simulink model "PID_controlinput"  (R2022a)
settings: Solver=VariableStepAuto  StartTime=0.0  StopTime=100  RelTol=1e-3
libraries: cstblocks x2
settings Model: Creator=Linxi Ren  LastModifiedBy=Linxi Ren

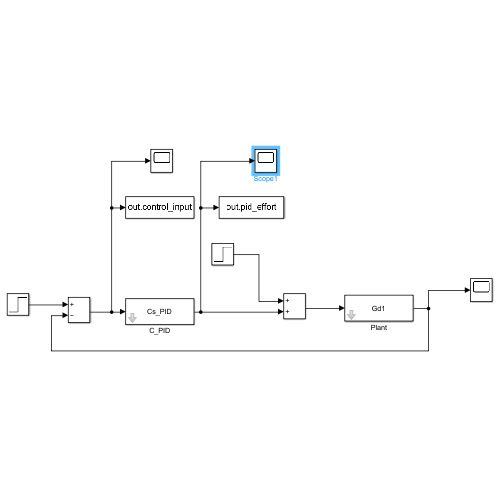
[thumbnail: Simulink's stored preview of the top-level diagram]
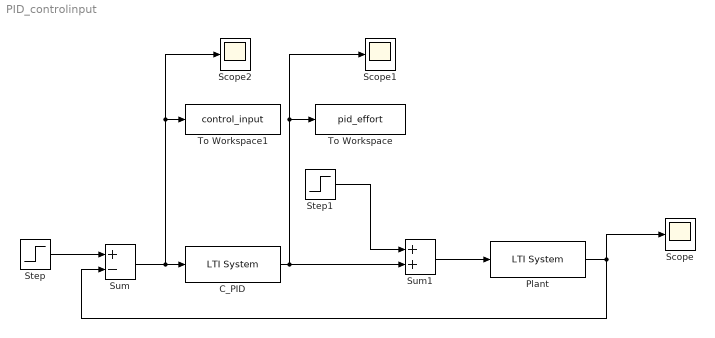
== system PID_controlinput ==
  C_PID : cstblocks/LTI System  sys=Cs_PID  IC=[]
  Plant : cstblocks/LTI System  sys=Gd1  IC=[]
  Scope : Scope
  Scope1 : Scope
  Scope2 : Scope
  Step : Step  Time=0  After=0  SampleTime=0
  Step1 : Step  Before=0.25  After=0.25  SampleTime=0
  Sum : Sum  Inputs=+-  InputSameDT=on  SaturateOnIntegerOverflow=on  OutDataTypeStr=Inherit: Same as first input
  Sum1 : Sum  InputSameDT=on  SaturateOnIntegerOverflow=on  OutDataTypeStr=Inherit: Same as first input
  To Workspace : ToWorkspace  VariableName=pid_effort  SaveFormat=Timeseries  SampleTime=-1
  To Workspace1 : ToWorkspace  VariableName=control_input  SaveFormat=Timeseries  SampleTime=-1
  wires:
  C_PID/1 -> Sum1/2, To Workspace/1, Scope1/1
  Plant/1 -> Sum/2, Scope/1
  Sum1/1 -> Plant/1
  Step/1 -> Sum/1
  Step1/1 -> Sum1/1
  Sum/1 -> Scope2/1, To Workspace1/1, C_PID/1
